simulink model "motor"  (R2017b)
settings: Solver=VariableStepAuto  StartTime=0.0  StopTime=10.0  RelTol=1e-3
settings Model: Creator=alinvoicu26  LastModifiedBy=alinvoicu26

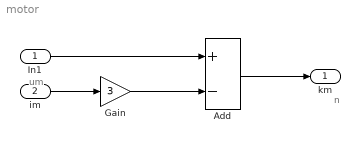
== system motor ==
  note: n
  note: um
  In1 : Inport
  "im " : Inport  Port=2
  Add : Sum  Inputs=+-
  Gain : Gain  Gain=3
  km : Outport
  wires:
  In1/1 -> Add/1
  "im "/1 -> Gain/1
  Gain/1 -> Add/2
  Add/1 -> km/1
